simulink model "workshop6_DCMotor_discretisedCtl"  (R2026a)
settings: Solver=VariableStepAuto  StopTime=0.5
values from neighbouring files (symbols this model uses):
  C = kp + ki/s + (kd*s)/(1+s*Tf)    [workshop6_deriv_setupParams.m]    (also in workshop6_discretisedCtl_setupParams.m = kd*s/(Tf*s+1) + kp + ki/s)
  Cd = c2d(C,Ts,'tustin')    [workshop6_discretisedCtl_setupParams.m]
  S_simple = (K/R)/(J*s+b+(K^2)/R)    [workshop6_deriv_setupParams.m]    (also in workshop6_discretisedCtl_setupParams.m)
  Ts = Trise/N    [workshop6_discretisedCtl_setupParams.m]
undefined symbols (not defined in the file or in its folder): dspblkCoreblockFVToolHelper, gcbh
libraries: simulink x1
settings Model: Creator=leoyi  LastModifiedBy=socks

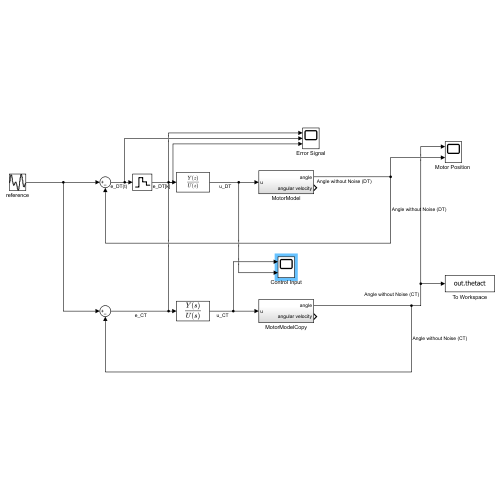
[thumbnail: Simulink's stored preview of the top-level diagram]
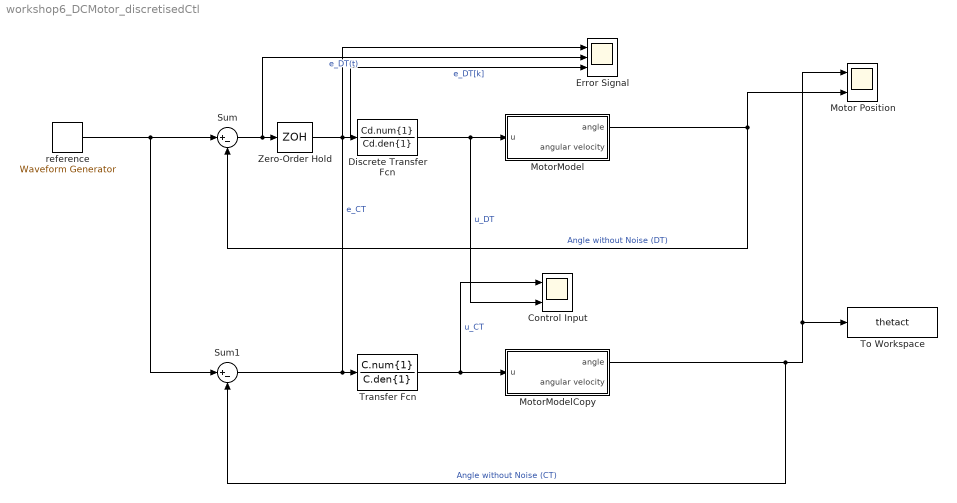
== system workshop6_DCMotor_discretisedCtl ==
  Control Input : Scope  NumInputPorts=2
      settings: ActiveDisplayYMinimum=-3.4450481984274197  ActiveDisplayYMaximum=5.0302522620159351  DataLoggingVariableName=ScopeData2
  Discrete Transfer Fcn : DiscreteTransferFcn  LoadFcn=dspblkCoreblockFVToolHelper(gcbh,'load');  Numerator=Cd.num{1}  Denominator=Cd.den{1}  SampleTime=Ts
      settings: CopyFcn=dspblkCoreblockFVToolHelper(gcbh,'copy');  DeleteFcn=dspblkCoreblockFVToolHelper(gcbh,'close');  ModelCloseFcn=dspblkCoreblockFVToolHelper(gcbh,'close');  PreSaveFcn=dspblkCoreblockFVToolHelper(gcbh,'presave');  PostSaveFcn=dspblkCoreblockFVToolHelper(gcbh,'postsave');  CloseFcn=dspblkCoreblockFVToolHelper(gcbh,'close');
  Error Signal : Scope  NumInputPorts=3
      settings: ActiveDisplayYMinimum=-0.60771  ActiveDisplayYMaximum=1.10991
  "Motor Position " : Scope  NumInputPorts=2
      settings: ActiveDisplayYMinimum=-0.14735  ActiveDisplayYMaximum=1.32614
  MotorModel : Subsystem
  MotorModelCopy : Subsystem
  Sum : Sum  Inputs=|+-
  Sum1 : Sum  Inputs=|+-
  To Workspace : ToWorkspace  VariableName=thetact  SaveFormat=Timeseries  SampleTime=-1
  Transfer Fcn : TransferFcn  Numerator=C.num{1}  Denominator=C.den{1}
  Zero-Order Hold : ZeroOrderHold  SampleTime=Ts
  reference : simulink/Sources/Waveform Generator  OutMin=[]  OutMax=[]  OutDataTypeStr=double  SelectedSignal=1  Signals=1#square('Amplitude',1,'Frequency',2*pi/0.25,'Phase',0,'DutyCycle',50)  BlockNames=MultiportSwitch_5740d72aaa054f2#MultiportSwitch_ba4dfc40e38844e  SampleTime=0.001
  wires:
  Discrete Transfer Fcn/1 -> Control Input/2, MotorModel/1(u)  "u_DT"
  reference/1 -> Sum1/1, Sum/1
  MotorModel/1(angle) -> "Motor Position "/2, Sum/2  "Angle without Noise (DT)"
  Sum/1 -> Error Signal/2, Zero-Order Hold/1  "e_DT(t)"
  Zero-Order Hold/1 -> Error Signal/3, Discrete Transfer Fcn/1  "e_DT[k]"
  Sum1/1 -> Error Signal/1, Transfer Fcn/1  "e_CT"
  MotorModelCopy/1(angle) -> "Motor Position "/1, To Workspace/1, Sum1/2  "Angle without Noise (CT)"
  Transfer Fcn/1 -> Control Input/1, MotorModelCopy/1(u)  "u_CT"

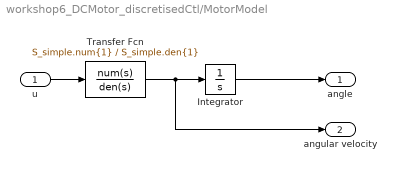
== system workshop6_DCMotor_discretisedCtl/MotorModel ==
  u : Inport
  Integrator : Integrator
  Transfer Fcn : TransferFcn  Numerator=S_simple.num{1}  Denominator=S_simple.den{1}
  angle : Outport
  angular velocity : Outport  Port=2
  wires:
  u/1 -> Transfer Fcn/1
  Transfer Fcn/1 -> angular velocity/1, Integrator/1
  Integrator/1 -> angle/1

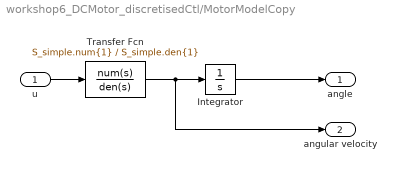
== system workshop6_DCMotor_discretisedCtl/MotorModelCopy ==
  u : Inport
  Integrator : Integrator
  Transfer Fcn : TransferFcn  Numerator=S_simple.num{1}  Denominator=S_simple.den{1}
  angle : Outport
  angular velocity : Outport  Port=2
  wires:
  u/1 -> Transfer Fcn/1
  Transfer Fcn/1 -> angular velocity/1, Integrator/1
  Integrator/1 -> angle/1
